simulink model "AM"  (R2020b)
settings: Solver=VariableStepAuto  StartTime=0.0  StopTime=10.0  RelTol=1e-3
settings Model: Creator=MEDIA  LastModifiedBy=MEDIA

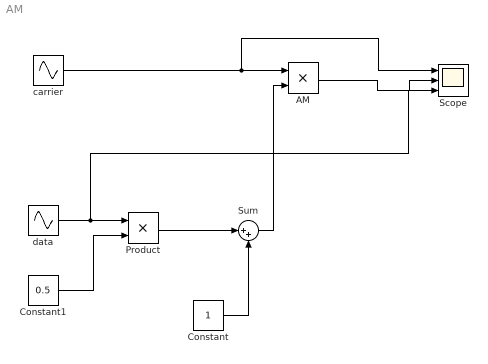
== system AM ==
  AM : Product
  Constant : Constant
  Constant1 : Constant  Value=0.5
  Product : Product
  Scope : Scope  NumInputPorts=3
  Sum : Sum  Inputs=|++
  carrier : Sin  Frequency=2*pi*25  SampleTime=1/5000
  data : Sin  Frequency=2*pi  SampleTime=1/5000
  wires:
  data/1 -> Scope/2, Product/1
  Constant1/1 -> Product/2
  Product/1 -> Sum/1
  Constant/1 -> Sum/2
  carrier/1 -> Scope/1, AM/1
  Sum/1 -> AM/2
  AM/1 -> Scope/3
